simulink model "matlab_test_environment_oldVersion"  (R2021b)
settings: Solver=VariableStepAuto  StartTime=0.0  StopTime=20.0  RelTol=1e-3  EnableMultiTasking=on
libraries: simulink_extras x2, simulink x1
settings Model: Creator=ndoehlert  LastModifiedBy=s140
settings SolverCC: ZeroCrossAlgorithm=Adaptive  AlgebraicLoopSolver=TrustRegion
settings DataIOCC: LimitDataPoints=on  ReturnWorkspaceOutputs=off
settings OptimizationCC: LifeSpan=inf
settings DebuggingCC: IgnoredZcDiagnostic=none  AllowSymbolicDim=off  SFUnexpectedBacktrackingDiag=warning  SFNoUnconditionalDefaultTransitionDiag=warning  SFExecutionAtInitializationDiag=none  SFMachineParentedDataDiag=warning  ArithmeticOperatorsInVariantConditions=warning
settings ModelReferenceCC: PropagateSignalLabelsOutOfModel=off
settings SFSimCC: SimUseLocalCustomCode=off  CustomCodeUndefinedFunction=UseInterfaceOnly
settings RTWCC: RTWUseLocalCustomCode=off
settings CodeAppCC: StateflowObjectComments=on
settings GRTTargetCC: TargetLangStandard=C89/C90 (ANSI)
settings ConfigComp: CovMetricSettings=dw  CovSaveCumulativeToWorkspaceVar=on  CovSaveSingleToWorkspaceVar=on  CovExternalEMLEnable=off

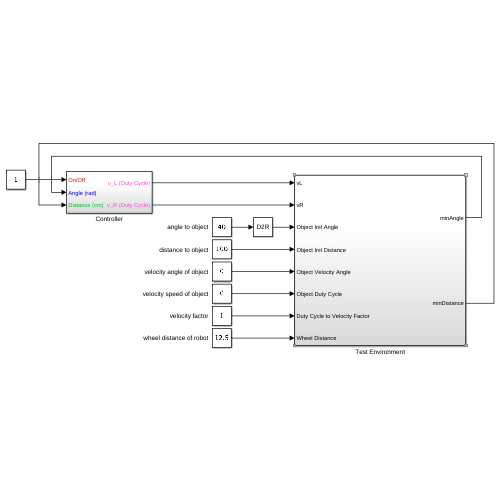
[thumbnail: Simulink's stored preview of the top-level diagram]
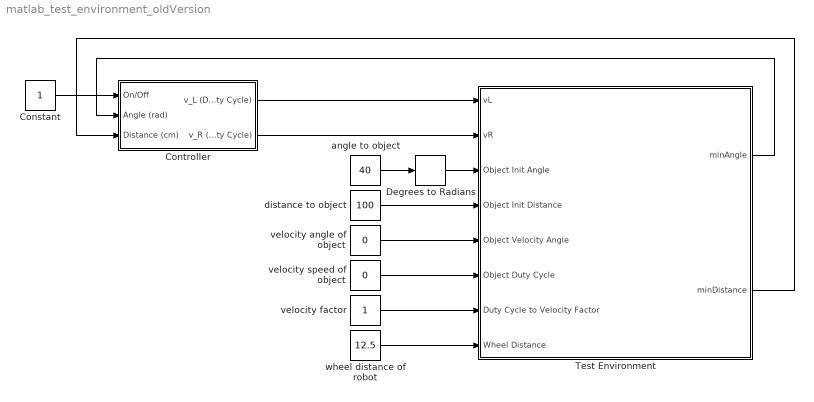
== system matlab_test_environment_oldVersion ==
  Constant : Constant
  Controller : Subsystem
  Degrees to Radians : simulink_extras/Transformations/Degrees to Radians
  Test Environment : Subsystem
  angle to object : Constant  Value=40
  distance to object : Constant  Value=100
  velocity angle of object : Constant  Value=0
  velocity factor : Constant
  velocity speed of object : Constant  Value=0
  wheel distance of robot : Constant  Value=12.5
  wires:
  Controller/1(v_L (Duty Cycle)) -> Test Environment/1(vL)
  Controller/2(v_R (Duty Cycle)) -> Test Environment/2(vR)
  Test Environment/2(minDistance) -> Controller/3(Distance (cm))
  Test Environment/1(minAngle) -> Controller/2(Angle (rad))
  angle to object/1 -> Degrees to Radians/1
  distance to object/1 -> Test Environment/4(Object Init Distance)
  velocity angle of object/1 -> Test Environment/5(Object Velocity Angle)
  velocity speed of object/1 -> Test Environment/6(Object Duty Cycle)
  velocity factor/1 -> Test Environment/7(Duty Cycle to Velocity Factor)
  wheel distance of robot/1 -> Test Environment/8(Wheel Distance)
  Degrees to Radians/1 -> Test Environment/3(Object Init Angle)
  Constant/1 -> Controller/1(On/Off)

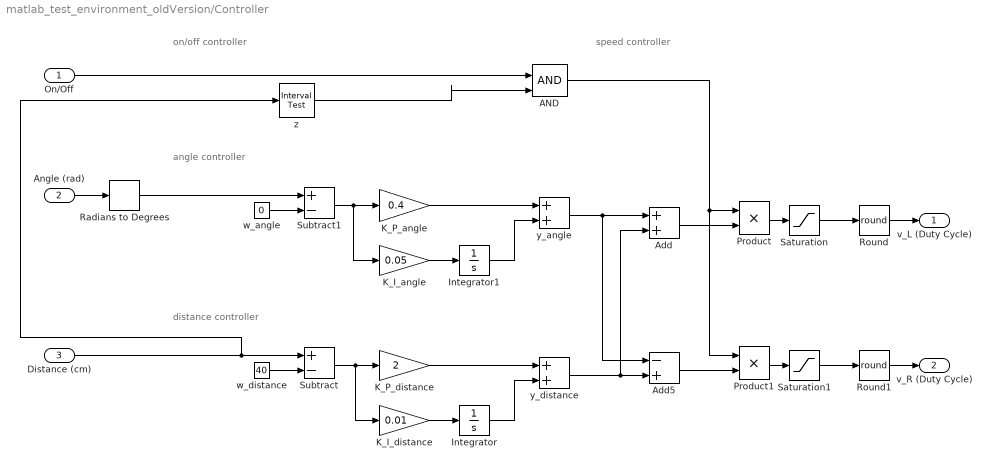
== system matlab_test_environment_oldVersion/Controller ==
  note: on/off controller
  note: angle controller
  note: distance controller
  note: speed controller
  On/Off : Inport
  Angle (rad) : Inport  Port=2
  Distance (cm) : Inport  Port=3
  AND : Logic  IconShape=distinctive  AllPortsSameDT=off  OutDataTypeStr=boolean
  Add : Sum
  Add5 : Sum  Inputs=-+
  Integrator : Integrator  LimitOutput=on  UpperSaturationLimit=200  LowerSaturationLimit=-200
  Integrator1 : Integrator  LimitOutput=on  UpperSaturationLimit=200  LowerSaturationLimit=-200
  K_I_angle : Gain  Gain=0.05
  K_I_distance : Gain  Gain=0.01
  K_P_angle : Gain  Gain=0.4
  K_P_distance : Gain  Gain=2
  Product : Product
  Product1 : Product
  Radians to Degrees : simulink_extras/Transformations/Radians to Degrees
  Round : Rounding  Operator=round
  Round1 : Rounding  Operator=round
  Saturation : Saturate  UpperLimit=100  LowerLimit=-100
  Saturation1 : Saturate  UpperLimit=100  LowerLimit=-100
  Subtract : Sum  Inputs=+-
  Subtract1 : Sum  Inputs=+-
  w_angle : Constant  Value=0
  w_distance : Constant  Value=40
  y_angle : Sum
  y_distance : Sum
  z : simulink/Logic and Bit Operations/Interval Test  IntervalClosedRight=on  uplimit=150  IntervalClosedLeft=on  lowlimit=25  OutDataTypeStr=boolean
  v_L (Duty Cycle) : Outport
  v_R (Duty Cycle) : Outport  Port=2
  wires:
  Angle (rad)/1 -> Radians to Degrees/1
  Round/1 -> v_L (Duty Cycle)/1
  Round1/1 -> v_R (Duty Cycle)/1
  Product1/1 -> Saturation1/1
  Radians to Degrees/1 -> Subtract1/1
  K_I_angle/1 -> Integrator1/1
  w_angle/1 -> Subtract1/2
  y_distance/1 -> Add/2, Add5/2
  K_I_distance/1 -> Integrator/1
  w_distance/1 -> Subtract/2
  AND/1 -> Product1/1, Product/1
  Product/1 -> Saturation/1
  Distance (cm)/1 -> z/1, Subtract/1
  Add/1 -> Product/2
  Subtract/1 -> K_P_distance/1, K_I_distance/1
  Subtract1/1 -> K_P_angle/1, K_I_angle/1
  Saturation/1 -> Round/1
  On/Off/1 -> AND/1
  Integrator1/1 -> y_angle/2
  y_angle/1 -> Add/1, Add5/1
  z/1 -> AND/2
  K_P_distance/1 -> y_distance/1
  Add5/1 -> Product1/2
  K_P_angle/1 -> y_angle/1
  Integrator/1 -> y_distance/2
  Saturation1/1 -> Round1/1

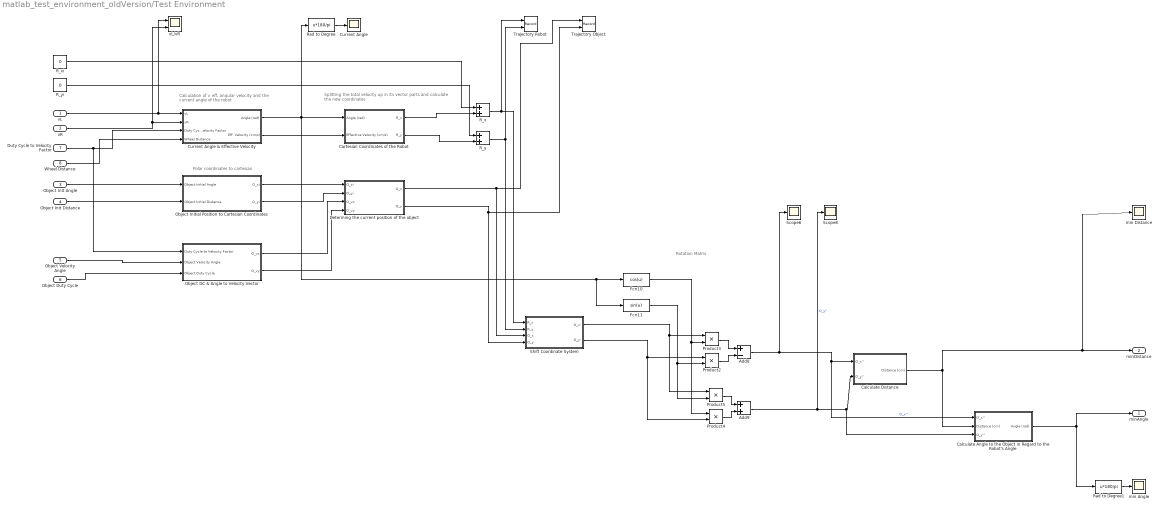
== system matlab_test_environment_oldVersion/Test Environment ==
  note: Splitting the total velocity up in its vector parts and calculate
      | the new coordinates
  note: Calculation of v_eff, angular velocity and the
      | current angle of the robot
  note: Rotation Matrix
  note: Polar coordinates to cartesian
  vL : Inport
  vR : Inport  Port=2
  Object Init Angle : Inport  Port=3
  Object Init Distance : Inport  Port=4
  Object Velocity Angle : Inport  Port=5
  Object Duty Cycle : Inport  Port=6
  Duty Cycle to Velocity Factor : Inport  Port=7
  Wheel Distance : Inport  Port=8
  Add8 : Sum  Inputs=+-
  Add9 : Sum
  Calculate Angle to the Object in Regard to the Robot's Angle : Subsystem
  Calculate Distance : Subsystem
  Cartesian Coordinates of the Robot : Subsystem
  Current Angle : Scope
  Current Angle & Effective Velocity : Subsystem
  Determing the current position of the object : Subsystem
  Fcn10 : Fcn  Expr=cos(u)
  Fcn11 : Fcn  Expr=sin(u)
  Object DC & Angle to Velocity Vector : Subsystem
  Object Initial Position to Cartesian Coordinates : Subsystem
  Product{2..5} (4 alike) : Product
  R_x : Sum
  R_xi : Constant  Value=0
  R_y : Sum
  R_yi : Constant  Value=0
  Rad to Degree : Fcn  Expr=u*180/pi
  Rad to Degree1 : Fcn  Expr=u*180/pi
  Scope6 : Scope
  Scope8 : Scope
  Shift Coordinate System : Subsystem
  Trajectory Object : Record  FileSettingsInternal="{\"entries\":[{\"content\":{\"excelSettings\":{\"content\":{},\"type\":\"Streamout.ExcelSettings\"}},\"type\":\"Streamout.FileSettingStorage\",\"uuid\":\"09e5390d-ee28-4a15-8892-7c9361f359b2\"}],\"packageUris\":[\"http://schema.mathworks.com/mf0/streamout_blocks/R2020a\"],\"version\":\"1.0\"}"  Layout=[1 1]  SignalsInternal="{\"entries\":[{\"content\":{\"signals\":[{\"content\":{\"blockPath\":[\"TestEnvironment/Test Environment/Trajectory Object\"],\"channel\":[],\"dimensions\":[1],\"domain\":\"TestEnvironment/Test Environment/Trajectory Object\",\"lineColor\":\"#a2142f\",\"plots\":[1],\"port\":1,\"sid\":[],\"signalID\":62,\"signalName\":\"Determing the current position of the object:1\"},\"type\":\"RecordBlkView.Signal\",\"uuid\":\"48eecbf5-aa71-433e-a936-a32114cb10b4\"},{\"content\":{\"blockPath\":[\"TestEnvironment/Test Environment/Trajectory Object\"],\"channel\":[],\"dimensions\":[1],\"domain\":\"TestEnvironment/Test Environment/Trajectory Object\",\"lineColor\":\"#139fff\",\"plots\":[1],\"port\":2,\"sid\":[],\"signalID\":65,\"signalName\":\"Determing the current position of the object:2\"},\"type\":\"RecordBlkView.Signal\",\"uuid\":\"78ec8a34-108b-4b9a-8c31-afffe5d0f788\"}]},\"type\":\"RecordBlkView.InputSignals\",\"uuid\":\"9307aaf4-76f8-4513-897a-10878db34b8a\"}],\"packageUris\":[\"http://schema.mathworks.com/mf0/streamout_blocks/R2020a\"],\"version\":\"1.0\"}"  VisualizationBindings="{\"xyplotplugin\":{\"info\":[{\"series\":[{\"bindingParametersList\":[{\"parameter\":\"X-Axis\",\"signalID\":62,\"signalName\":\"Determing the current position of the object:1\"},{\"parameter\":\"Y-Axis\",\"signalID\":65,\"signalName\":\"Determing the current position of the object:2\"}],\"seriesID\":21414}],\"subplotID\":1}]}}"  CompatibilityTag=XY  st=-1
  Trajectory Robot : Record  FileSettingsInternal="{\"entries\":[{\"content\":{\"excelSettings\":{\"content\":{},\"type\":\"Streamout.ExcelSettings\"}},\"type\":\"Streamout.FileSettingStorage\",\"uuid\":\"7d108c04-94ba-47e8-9fb1-e4674b5b2bbf\"}],\"packageUris\":[\"http://schema.mathworks.com/mf0/streamout_blocks/R2020a\"],\"version\":\"1.0\"}"  Layout=[1 1]  SignalsInternal="{\"entries\":[{\"content\":{\"signals\":[{\"content\":{\"blockPath\":[\"TestEnvironment/Test Environment/Trajectory Robot\"],\"channel\":[],\"dimensions\":[1],\"domain\":\"TestEnvironment/Test Environment/Trajectory Robot\",\"lineColor\":\"#a2142f\",\"plots\":[1],\"port\":1,\"sid\":[],\"signalID\":54,\"signalName\":\"R_x\"},\"type\":\"RecordBlkView.Signal\",\"uuid\":\"14a310e9-9ee9-49a3-a052-bc014900ea33\"},{\"content\":{\"blockPath\":[\"TestEnvironment/Test Environment/Trajectory Robot\"],\"channel\":[],\"dimensions\":[1],\"domain\":\"TestEnvironment/Test Environment/Trajectory Robot\",\"lineColor\":\"#139fff\",\"plots\":[1],\"port\":2,\"sid\":[],\"signalID\":57,\"signalName\":\"R_y\"},\"type\":\"RecordBlkView.Signal\",\"uuid\":\"d8f6eb97-e219-423b-ae19-e21060fa6ec9\"}]},\"type\":\"RecordBlkView.InputSignals\",\"uuid\":\"3fb910b1-0b5a-4e22-8f37-26dc61893521\"}],\"packageUris\":[\"http://schema.mathworks.com/mf0/streamout_blocks/R2020a\"],\"version\":\"1.0\"}"  VisualizationBindings="{\"xyplotplugin\":{\"info\":[{\"series\":[{\"bindingParametersList\":[{\"parameter\":\"X-Axis\",\"signalID\":54,\"signalName\":\"R_x\"},{\"parameter\":\"Y-Axis\",\"signalID\":57,\"signalName\":\"R_y\"}],\"seriesID\":44568}],\"subplotID\":1}]}}"  CompatibilityTag=XY  st=-1
  min Angle : Scope
  min Distance : Scope
  vL/vR : Scope  NumInputPorts=2
  minAngle : Outport
  minDistance : Outport  Port=2
  wires:
  vL/1 -> vL/vR/1, Current Angle & Effective Velocity/1(vL)
  vR/1 -> Current Angle & Effective Velocity/2(vR), vL/vR/2
  R_xi/1 -> R_x/1
  R_yi/1 -> R_y/1
  R_x/1 -> Shift Coordinate System/1(R_x), Trajectory Robot/1
  R_y/1 -> Shift Coordinate System/2(R_y), Trajectory Robot/2
  Duty Cycle to Velocity Factor/1 -> Current Angle & Effective Velocity/3(Duty Cycle to Velocity Factor), Object DC & Angle to Velocity Vector/1(Duty Cycle to Velocity Factor)
  Rad to Degree/1 -> Current Angle/1
  Fcn10/1 -> Product4/1, Product3/2
  Fcn11/1 -> Product5/2, Product2/2
  Product3/1 -> Add8/1
  Product2/1 -> Add8/2
  Product5/1 -> Add9/1
  Product4/1 -> Add9/2
  Add8/1 -> Calculate Angle to the Object in Regard to the Robot's Angle/1(O_x''), Calculate Distance/1(O_x''), Scope6/1  "O_x''"
  Add9/1 -> Calculate Angle to the Object in Regard to the Robot's Angle/3(O_y''), Calculate Distance/2(O_y''), Scope8/1  "O_y''"
  Rad to Degree1/1 -> min Angle/1
  Current Angle & Effective Velocity/1(Angle (rad)) -> Fcn11/1, Fcn10/1, Cartesian Coordinates of the Robot/1(Angle (rad)), Rad to Degree/1
  Wheel Distance/1 -> Current Angle & Effective Velocity/4(Wheel Distance)
  Current Angle & Effective Velocity/2(Eff. Velocity (cm/s)) -> Cartesian Coordinates of the Robot/2(Effective Velocity (cm/s))
  Cartesian Coordinates of the Robot/1(R_x) -> R_x/2
  Cartesian Coordinates of the Robot/2(R_y) -> R_y/2
  Object Init Angle/1 -> Object Initial Position to Cartesian Coordinates/1(Object Initial Angle)
  Object Init Distance/1 -> Object Initial Position to Cartesian Coordinates/2(Object Initial Distance)
  Object Velocity Angle/1 -> Object DC & Angle to Velocity Vector/2(Object Velocity Angle)
  Object Duty Cycle/1 -> Object DC & Angle to Velocity Vector/3(Object Duty Cycle)
  Determing the current position of the object/2(O_y) -> Shift Coordinate System/4(O_y), Trajectory Object/2
  Determing the current position of the object/1(O_x) -> Shift Coordinate System/3(O_x), Trajectory Object/1
  Object Initial Position to Cartesian Coordinates/1(O_xi) -> Determing the current position of the object/1(O_xi)
  Object Initial Position to Cartesian Coordinates/2(O_yi) -> Determing the current position of the object/2(O_yi)
  Object DC & Angle to Velocity Vector/1(O_vx) -> Determing the current position of the object/3(O_vx)
  Object DC & Angle to Velocity Vector/2(O_vy) -> Determing the current position of the object/4(O_vy)
  Shift Coordinate System/2(O_y') -> Product4/2, Product2/1
  Shift Coordinate System/1(O_x') -> Product5/1, Product3/1
  Calculate Distance/1(Distance (cm)) -> Calculate Angle to the Object in Regard to the Robot's Angle/2(Distance (cm)), min Distance/1, minDistance/1
  Calculate Angle to the Object in Regard to the Robot's Angle/1(Angle (rad)) -> minAngle/1, Rad to Degree1/1

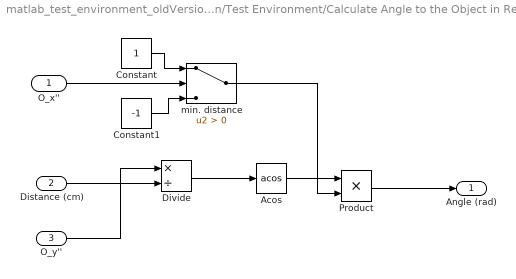
== system matlab_test_environment_oldVersion/Test Environment/Calculate Angle to the Object in Regard to the Robot's Angle ==
  O_x'' : Inport
  Distance (cm) : Inport  Port=2
  O_y'' : Inport  Port=3
  Acos : Trigonometry  Operator=acos
  Constant : Constant
  Constant1 : Constant  Value=-1
  Divide : Product  Inputs=*/
  Product : Product
  min. distance : Switch  Criteria=u2 > Threshold  ZeroCross=off
  Angle (rad) : Outport
  wires:
  Divide/1 -> Acos/1
  Acos/1 -> Product/1
  O_y''/1 -> Divide/1
  O_x''/1 -> min. distance/2
  Constant/1 -> min. distance/1
  Constant1/1 -> min. distance/3
  min. distance/1 -> Product/2
  Product/1 -> Angle (rad)/1
  Distance (cm)/1 -> Divide/2

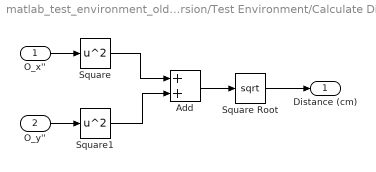
== system matlab_test_environment_oldVersion/Test Environment/Calculate Distance ==
  O_x'' : Inport
  O_y'' : Inport  Port=2
  Add : Sum
  Square : Math  Operator=square  SaturateOnIntegerOverflow=on
  Square Root : Sqrt  SaturateOnIntegerOverflow=on
  Square1 : Math  Operator=square  SaturateOnIntegerOverflow=on
  Distance (cm) : Outport
  wires:
  Square/1 -> Add/1
  Add/1 -> Square Root/1
  Square1/1 -> Add/2
  O_x''/1 -> Square/1
  O_y''/1 -> Square1/1
  Square Root/1 -> Distance (cm)/1

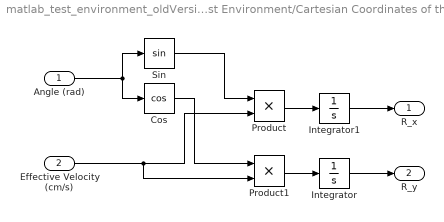
== system matlab_test_environment_oldVersion/Test Environment/Cartesian Coordinates of the Robot ==
  Angle (rad) : Inport
  Effective Velocity (cm/s) : Inport  Port=2
  Cos : Trigonometry  Operator=cos
  Integrator : Integrator
  Integrator1 : Integrator
  Product : Product
  Product1 : Product
  Sin : Trigonometry
  R_x : Outport
  R_y : Outport  Port=2
  wires:
  Angle (rad)/1 -> Cos/1, Sin/1
  Sin/1 -> Product/1
  Cos/1 -> Product1/1
  Effective Velocity (cm/s)/1 -> Product/2, Product1/2
  Product/1 -> Integrator1/1
  Product1/1 -> Integrator/1
  Integrator1/1 -> R_x/1
  Integrator/1 -> R_y/1

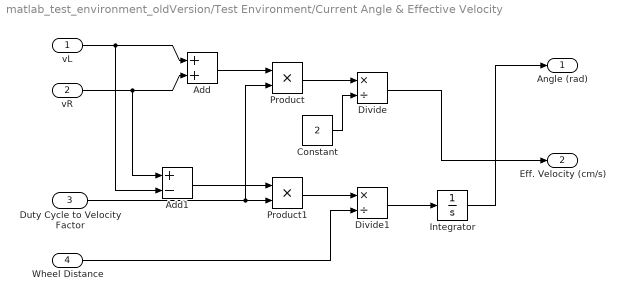
== system matlab_test_environment_oldVersion/Test Environment/Current Angle & Effective Velocity ==
  vL : Inport
  vR : Inport  Port=2
  Duty Cycle to Velocity Factor : Inport  Port=3
  Wheel Distance : Inport  Port=4
  Add : Sum
  Add1 : Sum  Inputs=+-
  Constant : Constant  Value=2
  Divide : Product  Inputs=*/
  Divide1 : Product  Inputs=*/
  Integrator : Integrator
  Product : Product
  Product1 : Product
  Angle (rad) : Outport
  Eff. Velocity (cm/s) : Outport  Port=2
  wires:
  Add/1 -> Product/1
  Product/1 -> Divide/1
  Constant/1 -> Divide/2
  Divide/1 -> Eff. Velocity (cm/s)/1
  Add1/1 -> Product1/1
  vR/1 -> Add1/1, Add/2
  Duty Cycle to Velocity Factor/1 -> Product1/2, Product/2
  vL/1 -> Add/1, Add1/2
  Product1/1 -> Divide1/1
  Wheel Distance/1 -> Divide1/2
  Divide1/1 -> Integrator/1
  Integrator/1 -> Angle (rad)/1

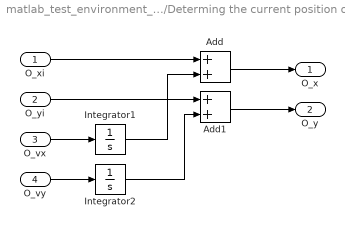
== system matlab_test_environment_oldVersion/Test Environment/Determing the current position of the object ==
  O_xi : Inport
  O_yi : Inport  Port=2
  O_vx : Inport  Port=3
  O_vy : Inport  Port=4
  Add : Sum
  Add1 : Sum
  Integrator1 : Integrator
  Integrator2 : Integrator
  O_x : Outport
  O_y : Outport  Port=2
  wires:
  O_xi/1 -> Add/1
  O_yi/1 -> Add1/1
  O_vx/1 -> Integrator1/1
  O_vy/1 -> Integrator2/1
  Integrator1/1 -> Add/2
  Integrator2/1 -> Add1/2
  Add/1 -> O_x/1
  Add1/1 -> O_y/1

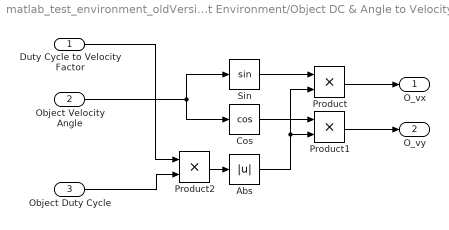
== system matlab_test_environment_oldVersion/Test Environment/Object DC & Angle to Velocity Vector ==
  Duty Cycle to Velocity Factor : Inport
  Object Velocity Angle : Inport  Port=2
  Object Duty Cycle : Inport  Port=3
  Abs : Abs
  Cos : Trigonometry  Operator=cos
  Product : Product
  Product1 : Product
  Product2 : Product
  Sin : Trigonometry
  O_vx : Outport
  O_vy : Outport  Port=2
  wires:
  Product/1 -> O_vx/1
  Product1/1 -> O_vy/1
  Abs/1 -> Product1/2, Product/2
  Sin/1 -> Product/1
  Object Velocity Angle/1 -> Cos/1, Sin/1
  Cos/1 -> Product1/1
  Duty Cycle to Velocity Factor/1 -> Product2/1
  Object Duty Cycle/1 -> Product2/2
  Product2/1 -> Abs/1

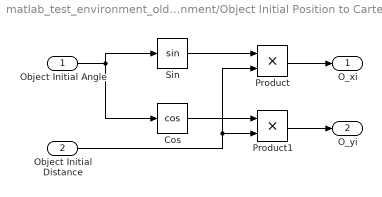
== system matlab_test_environment_oldVersion/Test Environment/Object Initial Position to Cartesian Coordinates ==
  Object Initial Angle : Inport
  Object Initial Distance : Inport  Port=2
  Cos : Trigonometry  Operator=cos
  Product : Product
  Product1 : Product
  Sin : Trigonometry
  O_xi : Outport
  O_yi : Outport  Port=2
  wires:
  Object Initial Angle/1 -> Cos/1, Sin/1
  Sin/1 -> Product/1
  Cos/1 -> Product1/1
  Object Initial Distance/1 -> Product1/2, Product/2
  Product/1 -> O_xi/1
  Product1/1 -> O_yi/1

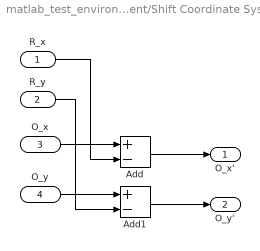
== system matlab_test_environment_oldVersion/Test Environment/Shift Coordinate System ==
  R_x : Inport
  R_y : Inport  Port=2
  O_x : Inport  Port=3
  O_y : Inport  Port=4
  Add : Sum  Inputs=+-
  Add1 : Sum  Inputs=+-
  O_x' : Outport
  O_y' : Outport  Port=2
  wires:
  O_x/1 -> Add/1
  O_y/1 -> Add1/1
  R_x/1 -> Add/2
  R_y/1 -> Add1/2
  Add/1 -> O_x'/1
  Add1/1 -> O_y'/1
